simulink model "SixStep_Hall_Simulation"  (R2024a)
settings: Solver=FixedStepAuto  StartTime=0.0  StopTime=10.0  FixedStep=1e-3  RelTol=1e-3
libraries: fuzblock x1
settings Model: Creator=18283  LastModifiedBy=18283

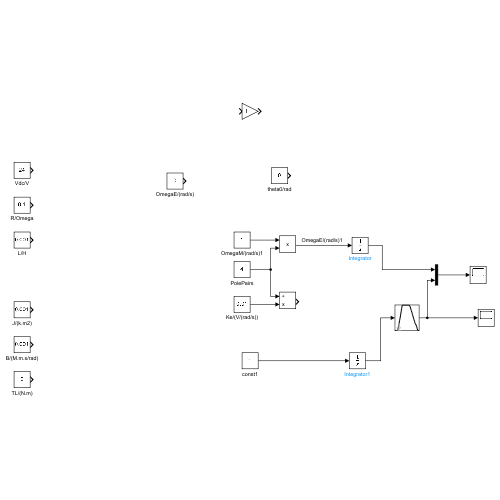
[thumbnail: Simulink's stored preview of the top-level diagram]
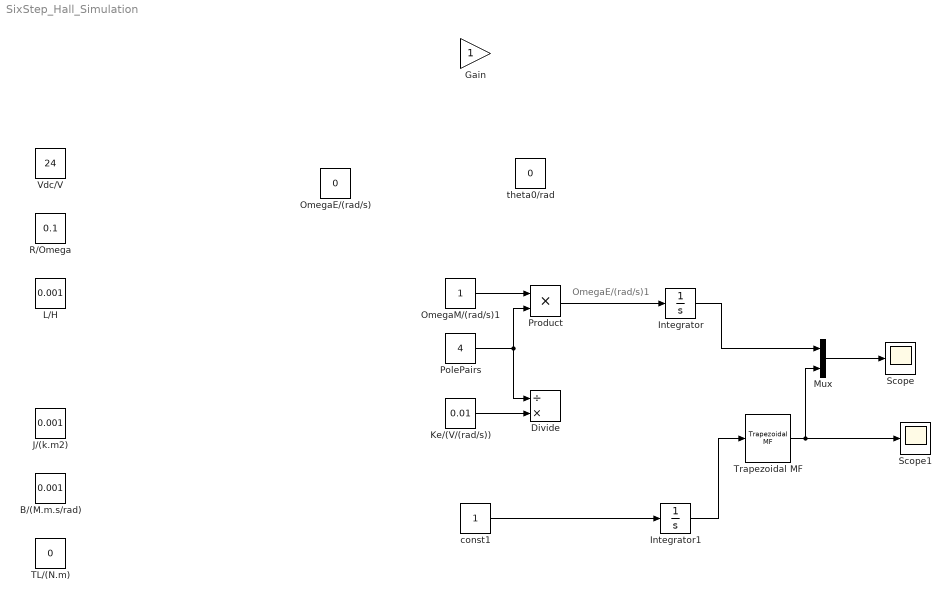
== system SixStep_Hall_Simulation ==
  note: OmegaE/(rad/s)1
  B/(M.m.s/rad) : Constant  Value=0.001
  Divide : Product  Inputs=/*
  Gain : Gain
  Integrator : Integrator
  Integrator1 : Integrator
  J/(k.m2) : Constant  Value=0.001
  Ke/(V/(rad/s)) : Constant  Value=0.01
  L/H : Constant  Value=0.001
  Mux : Mux  Inputs=2
  OmegaE/(rad/s) : Constant  Value=0
  OmegaM/(rad/s)1 : Constant
  PolePairs : Constant  Value=4
  Product : Product
  R/Omega : Constant  Value=0.1
  Scope : Scope
  Scope1 : Scope
  TL/(N.m) : Constant  Value=0
  Trapezoidal MF : fuzblock/Membership  Functions/Trapezoidal MF  a=1  b=5  c=7  d=8
  Vdc/V : Constant  Value=24
  const1 : Constant
  theta0/rad : Constant  Value=0
  wires:
  OmegaM/(rad/s)1/1 -> Product/1
  PolePairs/1 -> Divide/1, Product/2
  Product/1 -> Integrator/1
  Ke/(V/(rad/s))/1 -> Divide/2
  Trapezoidal MF/1 -> Scope1/1, Mux/2
  Integrator/1 -> Mux/1
  Mux/1 -> Scope/1
  const1/1 -> Integrator1/1
  Integrator1/1 -> Trapezoidal MF/1
